simulink model "c1_waypoint"  (R2021b)
settings: Solver=FixedStepDiscrete  StartTime=0.0  StopTime=Inf  FixedStep=sampleTime  RelTol=1e-3  EnableMultiTasking=on
InitFcn:
  | sampleTime = 0.05;
  | nMedianSize=3;
  | % Robot parameters
  | wheelRadius = 0.0303;
  | robotRadius = 0.06;   %小车在仿真中显示的圆形的半径大小
  | Trackwidth = 0.0847;  %定义向量场直方图算法中小车的宽度
  | 
  | % Lidar parameters
  | sensorOffset = [0,0];
  | scanAngles = linspace(-pi/2,pi/2,9)';
  | maxRange = 5;
  | 
  | %%%%%%
  | ks=1;
  | 
  | %初始位置
  | x_1_0=1;
  | y_1_0=1;
  | yaw_1_0=pi/4;
  | 
  | x_2_0=0;
  | y_2_0=0.3;
  | yaw_2_0=0;
  | 
  | x_3_0=0;
  | y_3_0=0.6;
  | yaw_3_0=0;
  | 
  | x_4_0=0;
  | y_4_0=0.9;
  | yaw_4_0=0;
  | 
  | 
  | A=0.3;
  | C=1.7;
  | B=(A+C)/2;
  | 
  | wp1=[A,A; B,A;  C,A; C,B;C,C; B,C; A,C;A,B];
  | WAY_P=[wp1;wp1;wp1;wp1];
undefined symbols (not defined in the file): Angular, DiscIntNeverNeededParam, Linear
libraries: robotlib x4, dspstat3 x3
settings Model: Creator=The MathWorks, Inc.  LastModifiedBy=FCS
settings SolverCC: AlgebraicLoopSolver=TrustRegion
settings DataIOCC: LimitDataPoints=on  SaveFormat=Array  ReturnWorkspaceOutputs=off
settings OptimizationCC: EnhancedBackFolding=on  PassReuseOutputArgsAs=Individual arguments  ZeroExternalMemoryAtStartup=off  ZeroInternalMemoryAtStartup=off  MaxStackSize=64  OptimizeBlockOrder=speed  DifferentSizesBufferReuse=on  OptimizationCustomize=off  EfficientTunableParamExpr=on
settings DebuggingCC: SolverPrmCheckMsg=warning  ParameterTunabilityLossMsg=error  SFUnexpectedBacktrackingDiag=warning  SFNoUnconditionalDefaultTransitionDiag=warning  SFExecutionAtInitializationDiag=none  SFMachineParentedDataDiag=warning  ArithmeticOperatorsInVariantConditions=warning
settings HardwareCC: ProdBitPerPointer=32  ProdBitPerSizeT=32  ProdBitPerPtrDiffT=32  ProdLargestAtomicFloat=None  ProdIntDivRoundTo=Undefined  ProdEndianess=Unspecified  ProdWordSize=32  ProdHWDeviceType=Generic->Unspecified (assume 32-bit Generic)  TargetHWDeviceType=Generic->Unspecified (assume 32-bit Generic)
settings ModelReferenceCC: PropagateSignalLabelsOutOfModel=off
settings SFSimCC: SimUseLocalCustomCode=off  MATLABDynamicMemAlloc=off  CustomCodeUndefinedFunction=UseInterfaceOnly  SimTargetLang=C++
settings RTWCC: Description=Embedded Coder  SystemTargetFile=ert.tlc  HardwareBoard=Robot Operating System (ROS)  TLCOptions="-aInlineSetEventsForThisBaseRateFcn=TLC_FALSE -aSuppressMultiTaskScheduler=TLC_FALSE  -aRateBasedStepFcn=0"  TemplateMakefile=ert_default_tmf  RTWUseLocalCustomCode=off  Toolchain=Catkin  TargetLang=C++
settings CodeAppCC: ForceParamTrailComments=on  IgnoreCustomStorageClasses=off  OperatorAnnotations=on  SimulinkDataObjDesc=on  SFDataObjDesc=on  InsertBlockDesc=on
settings ERTTargetCC: SupportVariableSizeSignals=on
settings ConfigComp: CovMetricSettings=dw  CovSaveCumulativeToWorkspaceVar=on  CovSaveSingleToWorkspaceVar=on  CovExternalEMLEnable=off  CovSFcnEnable=off

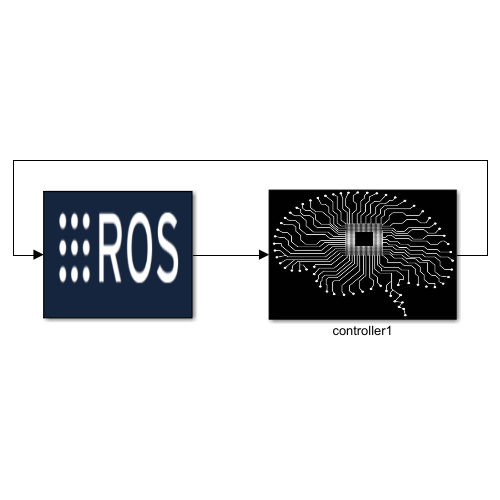
[thumbnail: Simulink's stored preview of the top-level diagram]
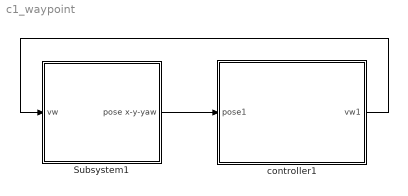
== system c1_waypoint ==
  Subsystem1 : Subsystem
      mask Display: image('$imagefile'); % 使用工具条上的 "编辑图像" 进行更改。
  controller1 : Subsystem
      mask Display: image('$imagefile'); % 使用工具条上的 "编辑图像" 进行更改。
  wires:
  controller1/1(vw1) -> Subsystem1/1(vw)
  Subsystem1/1(pose x-y-yaw) -> controller1/1(pose1)

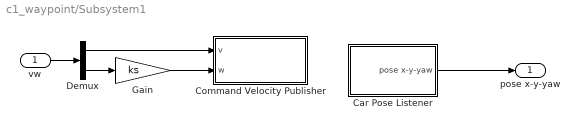
== system c1_waypoint/Subsystem1 ==
  vw : Inport
  Car Pose Listener : Subsystem
  Command Velocity Publisher : Subsystem
  Demux : Demux  Outputs=2
  Gain : Gain  Gain=ks
  pose x-y-yaw : Outport
  wires:
  Gain/1 -> Command Velocity Publisher/2(w)
  Demux/1 -> Command Velocity Publisher/1(v)
  vw/1 -> Demux/1
  Car Pose Listener/1(pose x-y-yaw) -> pose x-y-yaw/1
  Demux/2 -> Gain/1

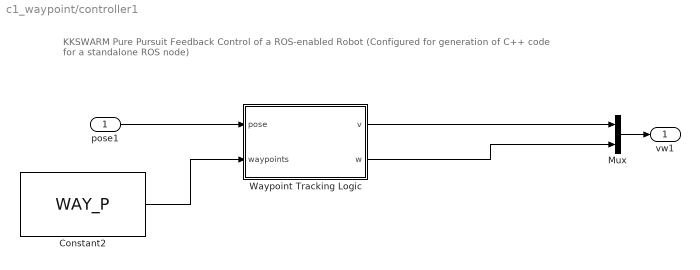
== system c1_waypoint/controller1 ==
  note: KKSWARM Pure Pursuit Feedback Control of a ROS-enabled Robot
      | (Configured for generation of C++ code for a standalone ROS node)
  pose1 : Inport
  Constant2 : Constant  Value=WAY_P
  Mux : Mux  Inputs=2
  Waypoint Tracking Logic : Stateflow chart  TreatAsAtomicUnit=on
  vw1 : Outport
  wires:
  Waypoint Tracking Logic/1(v) -> Mux/1
  pose1/1 -> Waypoint Tracking Logic/1(pose)
  Mux/1 -> vw1/1
  Waypoint Tracking Logic/2(w) -> Mux/2
  Constant2/1 -> Waypoint Tracking Logic/2(waypoints)

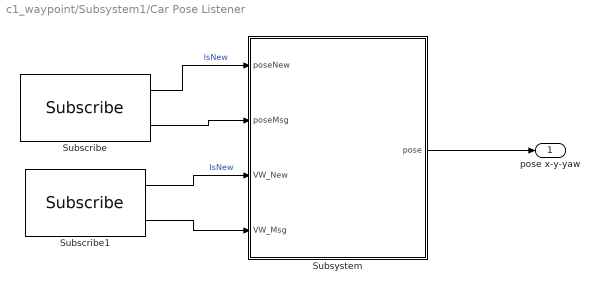
== system c1_waypoint/Subsystem1/Car Pose Listener ==
  Subscribe : robotlib/Subscribe  topicSource=Specify your own  topic=/robot_1/pose  messageType=nav_msgs/Odometry  SampleTime=-1  legacyBusStruct=off  messageQueueLength=51
  Subscribe1 : robotlib/Subscribe  topicSource=Specify your own  topic=/robot_1/odometry  messageType=geometry_msgs/Twist  SampleTime=-1  legacyBusStruct=off  messageQueueLength=51
  Subsystem : Subsystem
  pose x-y-yaw : Outport
  wires:
  Subscribe/1 -> Subsystem/1(poseNew)  "IsNew"
  Subscribe/2 -> Subsystem/2(poseMsg)
  Subscribe1/1 -> Subsystem/3(VW_New)  "IsNew"
  Subscribe1/2 -> Subsystem/4(VW_Msg)
  Subsystem/1(pose) -> pose x-y-yaw/1

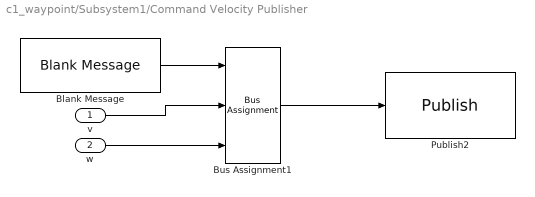
== system c1_waypoint/Subsystem1/Command Velocity Publisher ==
  v : Inport
  w : Inport  Port=2
  Blank Message : robotlib/Blank Message  messageClass=Message  entityType=geometry_msgs/Twist  messageType=geometry_msgs/Twist  SampleTime=inf  legacyBusStruct=off
  Bus Assignment1 : BusAssignment  DialogController=Simulink.DDGSource_BusAssignment  AssignedSignals=Linear.X,Angular.Z
  Publish2 : robotlib/Publish  topicSource=Specify your own  topic=/robot_1/cmd_vel  messageType=geometry_msgs/Twist  legacyBusStruct=off  messageQueueLength=105
  wires:
  Bus Assignment1/1 -> Publish2/1
  Blank Message/1 -> Bus Assignment1/1
  v/1 -> Bus Assignment1/2
  w/1 -> Bus Assignment1/3

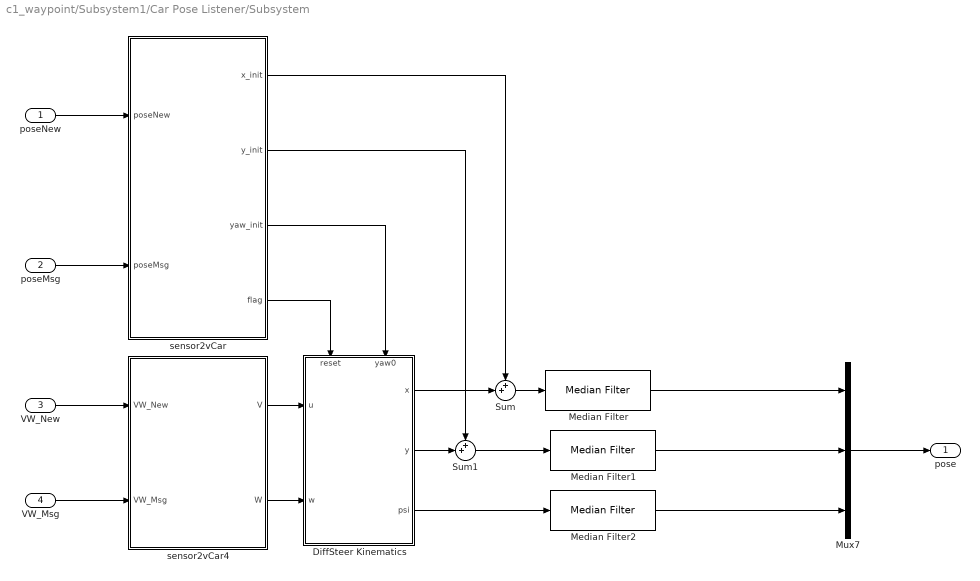
== system c1_waypoint/Subsystem1/Car Pose Listener/Subsystem ==
  poseNew : Inport
  poseMsg : Inport  Port=2
  VW_New : Inport  Port=3
  VW_Msg : Inport  Port=4
  DiffSteer Kinematics : Subsystem
      settings: PortSchema="{\"entries\":[{\"content\":{\"sides\":[{\"content\":{\"connectorIds\":[\"In1\",\"In2\"]},\"type\":\"ConnectorPlacement.EquallySpacedRectSide\",\"uuid\":\"0032ed68-1de4-4b1c-b237-9372fedc8a7a\"},{\"content\":{\"connectorIds\":[\"Out1\",\"Out2\",\"Out3\"],\"side\":\"RIGHT\"},\"type\":\"ConnectorPlacement.EquallySpacedRectSide\",\"uuid\":\"d0c861bd-7497-47fe-b183-36da470ee2c6\"},{\"content\":{\"connectorIds\":[\"In3\",\"In4\"],\"side\":\"TOP\"},\"type\":\"ConnectorPlacement.EquallySpacedRectSide\",\"uuid\":\"5b685229-150b-4cb5-b33d-c61d28c4627e\"}]},\"type\":\"ConnectorPlacement.EquallySpacedConnector\",\"uuid\":\"4513c50b-5820-40cb-bb28-cc7c1b1322fe\"}],\"packageUris\":[\"http://schema.mathworks.com/mf0/Connector/R2020b\"],\"version\":\"1.0\"}"
  Median Filter : dspstat3/Median Filter  WindowLength=nMedianSize  SimulateUsing=Interpreted execution
      settings: SourceProductBaseCode=DS
  Median Filter1 : dspstat3/Median Filter  WindowLength=nMedianSize  SimulateUsing=Interpreted execution
      settings: SourceProductBaseCode=DS
  Median Filter2 : dspstat3/Median Filter  WindowLength=nMedianSize  SimulateUsing=Interpreted execution
      settings: SourceProductBaseCode=DS
  Mux7 : Mux  Inputs=3
  Sum : Sum  Inputs=++|
  Sum1 : Sum  Inputs=++|
  sensor2vCar : MATLAB Function  TreatAsAtomicUnit=on
  sensor2vCar4 : MATLAB Function  TreatAsAtomicUnit=on
  pose : Outport
  wires:
  Median Filter2/1 -> Mux7/3
  Median Filter1/1 -> Mux7/2
  Median Filter/1 -> Mux7/1
  sensor2vCar/4(flag) -> DiffSteer Kinematics/3(reset)
  DiffSteer Kinematics/2(y) -> Sum1/2
  sensor2vCar/3(yaw_init) -> DiffSteer Kinematics/4(yaw0)
  sensor2vCar/2(y_init) -> Sum1/1
  sensor2vCar/1(x_init) -> Sum/1
  DiffSteer Kinematics/1(x) -> Sum/2
  VW_New/1 -> sensor2vCar4/1(VW_New)
  Mux7/1 -> pose/1
  Sum/1 -> Median Filter/1
  DiffSteer Kinematics/3(psi) -> Median Filter2/1
  sensor2vCar4/1(V) -> DiffSteer Kinematics/1(u)
  Sum1/1 -> Median Filter1/1
  sensor2vCar4/2(W) -> DiffSteer Kinematics/2(w)
  poseNew/1 -> sensor2vCar/1(poseNew)
  poseMsg/1 -> sensor2vCar/2(poseMsg)
  VW_Msg/1 -> sensor2vCar4/2(VW_Msg)

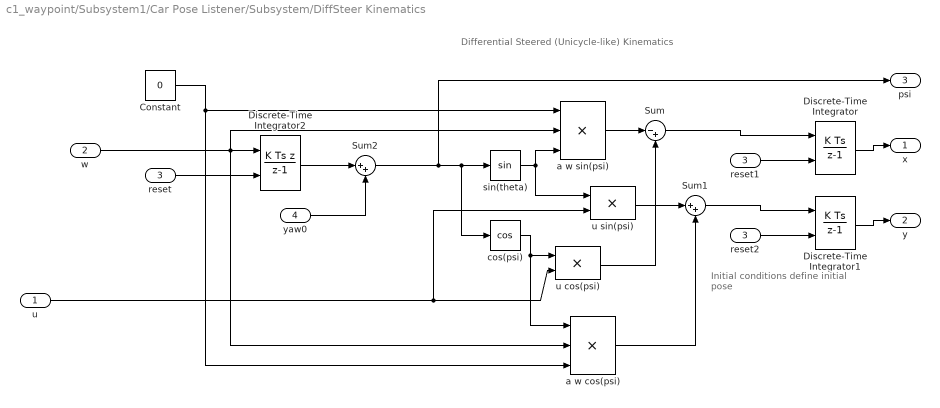
== system c1_waypoint/Subsystem1/Car Pose Listener/Subsystem/DiffSteer Kinematics ==
  note: Initial conditions define
      | initial pose
  note: Differential Steered (Unicycle-like) Kinematics
  u : Inport
  w : Inport  Port=2
  reset : Inport  Port=3
  yaw0 : Inport  Port=4
  Constant : Constant  Value=0
  Discrete-Time Integrator : DiscreteIntegrator  ExternalReset=falling  SampleTime=-1  ICPrevOutput=DiscIntNeverNeededParam  ICPrevScaledInput=DiscIntNeverNeededParam
  Discrete-Time Integrator1 : DiscreteIntegrator  ExternalReset=falling  SampleTime=-1  ICPrevOutput=DiscIntNeverNeededParam  ICPrevScaledInput=DiscIntNeverNeededParam
  Discrete-Time Integrator2 : DiscreteIntegrator  IntegratorMethod=Integration: Backward Euler  ExternalReset=falling  SampleTime=-1  ICPrevOutput=DiscIntNeverNeededParam  ICPrevScaledInput=DiscIntNeverNeededParam
  Sum : Sum  Inputs=|-+  SaturateOnIntegerOverflow=on
  Sum1 : Sum  Inputs=|++  SaturateOnIntegerOverflow=on
  Sum2 : Sum  Inputs=|++
  a w cos(psi) : Product  Inputs=3  SaturateOnIntegerOverflow=on  OutDataTypeStr=Inherit: Same as first input
  a w sin(psi) : Product  Inputs=3  SaturateOnIntegerOverflow=on  OutDataTypeStr=Inherit: Same as first input
  cos(psi) : Trigonometry  Operator=cos
  reset1 : InportShadow  Port=3
  reset2 : InportShadow  Port=3
  sin(theta) : Trigonometry
  u cos(psi) : Product  SaturateOnIntegerOverflow=on  OutDataTypeStr=Inherit: Same as first input
  u sin(psi) : Product  SaturateOnIntegerOverflow=on  OutDataTypeStr=Inherit: Same as first input
  x : Outport
  y : Outport  Port=2
  psi : Outport  Port=3
  wires:
  yaw0/1 -> Sum2/2
  reset2/1 -> Discrete-Time Integrator1/2
  reset1/1 -> Discrete-Time Integrator/2
  reset/1 -> Discrete-Time Integrator2/2
  u sin(psi)/1 -> Sum1/1
  cos(psi)/1 -> u cos(psi)/1, a w cos(psi)/1
  w/1 -> a w cos(psi)/2, a w sin(psi)/2, Discrete-Time Integrator2/1
  Constant/1 -> a w sin(psi)/1, a w cos(psi)/3
  Discrete-Time Integrator/1 -> x/1
  Sum/1 -> Discrete-Time Integrator/1
  sin(theta)/1 -> a w sin(psi)/3, u sin(psi)/1
  a w cos(psi)/1 -> Sum1/2
  Sum2/1 -> psi/1, sin(theta)/1, cos(psi)/1
  u cos(psi)/1 -> Sum/2
  u/1 -> u sin(psi)/2, u cos(psi)/2
  a w sin(psi)/1 -> Sum/1
  Sum1/1 -> Discrete-Time Integrator1/1
  Discrete-Time Integrator1/1 -> y/1
  Discrete-Time Integrator2/1 -> Sum2/1

== stateflow chart c1_waypoint/controller1/Waypoint Tracking Logic ==
  state FollowWaypoints
    entry:
    goalPoint = waypoints(idx,:);
    entry, during:
    [angle,range] = trackGoal(goalPoint);
    (default) -> (junction 20)
    FollowWaypoints -> (junction 20) [order 1]
    (junction 20) -> (junction 24) [order 1] : % Set angular speed if
        | % angle outside deadband
        | [abs(angle) > pi/24]
    (junction 20) -> (junction 30) [order 2] : {w = 0;}
    (junction 24) -> (junction 49) : % Proportional
        | % control
        | {w = 1.5*angle;}
    (junction 49) -> (junction 30)
  state ReachedGoal
    entry:
    v = 0;
    w = 0.5;
  (default) -> FollowWaypoints : {
      | v = 0.2;
      | idx = 1;
      | numPts = size(waypoints,1);
      | }
  FollowWaypoints -> (junction 39) [order 1] : % Check if goal reached
      | [range < 0.2]
  (junction 39) -> ReachedGoal [order 1] : % Stop if final waypoint
      | [idx == numPts]
  (junction 39) -> (junction 42) [order 2]
  (junction 42) -> FollowWaypoints : % Go to the next waypoint
      | {idx = idx + 1;}
  data: goal function_input; ang function_output; dist function_output; pose input; waypoints input; v output; w output; angle local; range local; idx local; numPts local; goalPoint local
  function [ang,dist] = trackGoal(goal):
    | function [ang,dist] = trackGoal(goal)
    | % Finds the angle (theta) and distance (dist) between the 
    | % vehicle and a goal point
    |     
    | posDiff = [goal(1)-pose(1);goal(2)-pose(2)];
    | 
    | ang = angdiff(pose(3),atan2(posDiff(2),posDiff(1)));
    | dist = sqrt(posDiff(1)^2 + posDiff(2)^2);

== matlab function c1_waypoint/Subsystem1/Car Pose Listener/Subsystem/sensor2vCar ==
  data: x_init output; y_init output; yaw_init output; flag output; poseNew input; poseMsg input
function [x_init,y_init,yaw_init,flag] = sensor2vCar(poseNew, poseMsg)
persistent x0 y0 yaw0 yaw1 x0_init y0_init yaw0_init fStart
if isempty(x0)
    x0=-10; y0=-10; yaw0=0; yaw1=0;   
    x0_init=-10;y0_init=-10;yaw0_init=0;
    fStart=0;
end
if poseNew
    if x0==poseMsg.Pose.Pose.Position.X&&y0==poseMsg.Pose.Pose.Position.Y
        flag=1;
    else
        x0=poseMsg.Pose.Pose.Position.X;
        y0=poseMsg.Pose.Pose.Position.Y;   
        %yaw2=atan2(2*(poseMsg.Pose.Pose.Orientation.Z*poseMsg.Pose.Pose.Orientation.W),1-2*(poseMsg.Pose.Pose.Orientation.Z^2)); 
        eul=quat2eul([poseMsg.Pose.Pose.Orientation.W,poseMsg.Pose.Pose.Orientation.X,poseMsg.Pose.Pose.Orientation.Y,poseMsg.Pose.Pose.Orientation.Z]);
        yaw2=eul(1);
        %对前后角度差使用积分，恢复yaw的连续性
        yaw0=yaw0+angdiff(yaw1,yaw2);
        yaw1=yaw2;
        flag=0;        
        x0_init=x0;
        y0_init=y0;
        yaw0_init=yaw0;
        fStart=1;
    end 
else
    if fStart
        flag=1;
    else
        flag=0;
    end
end

x_init=x0_init;y_init=y0_init;yaw_init=yaw0_init;

== matlab function c1_waypoint/Subsystem1/Car Pose Listener/Subsystem/sensor2vCar4 ==
  data: V output; W output; VW_New input; VW_Msg input
function [V,W] = sensor2vCar(VW_New, VW_Msg)
persistent v0 w0
if isempty(v0)
    v0=0; 
    w0=0;    
end
if VW_New
    v0=VW_Msg.Linear.X;
    w0=VW_Msg.Angular.Z;
end

V=v0;
W=-w0;
